simulink model "mcp4562"  (R2023b)
settings: Solver=VariableStepAuto  StartTime=0.0  StopTime=30  RelTol=1e-3
libraries: fl_lib x5, nesl_utility x3, ee_lib x1
settings Model: Creator=samuels  LastModifiedBy=samuels

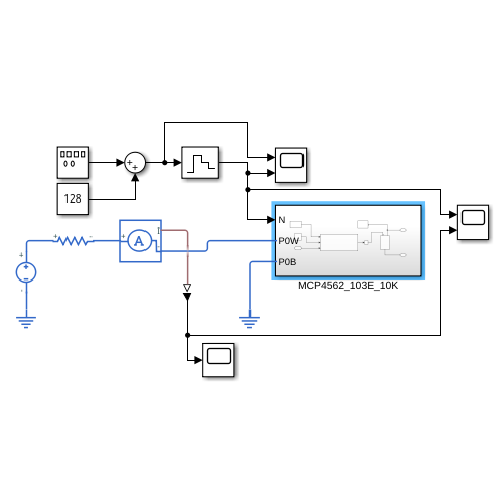
[thumbnail: Simulink's stored preview of the top-level diagram]
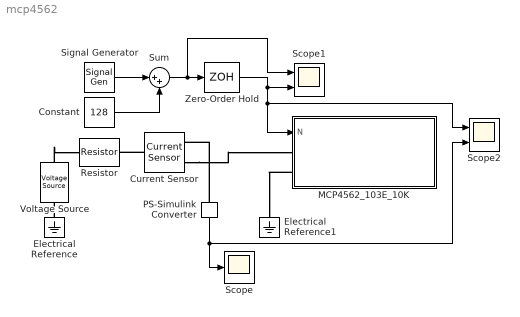
== system mcp4562 ==
  Constant : Constant  Value=128
  Current Sensor : fl_lib/Electrical/Electrical Sensors/Current Sensor
  Electrical Reference : fl_lib/Electrical/Electrical Elements/Electrical Reference
  Electrical Reference1 : fl_lib/Electrical/Electrical Elements/Electrical Reference
  MCP4562_103E_10K : Subsystem
  PS-Simulink Converter : nesl_utility/PS-Simulink Converter  PhysicalDomain=network_engine_domain  SubClassName=ps_output  LeftPortType=input  RightPortType=output  PseudoPeriodic=off  Frequencies=[]  VectorFormat=inherit  Unit=inherit  AffineConversion=off
  Resistor : fl_lib/Electrical/Electrical Elements/Resistor  R=100 Ohm  i_specify=off  i_priority=None  i=0 A  i_nominal_specify=off  i_nominal_unit=A  i_nominal_value=1  v_specify=off  v_priority=None  v=0 V  v_nominal_specify=off  v_nominal_unit=V  v_nominal_value=1
  Scope : Scope
  Scope1 : Scope  NumInputPorts=2
  Scope2 : Scope  NumInputPorts=2
  Signal Generator : SignalGenerator  WaveForm=sawtooth  Amplitude=128  Frequency=0.1
  Sum : Sum  Inputs=|++
  Voltage Source : ee_lib/Sources/Voltage Source  dc_voltage=1000 V  ac_voltage=0 V  ac_shift=0 rad  ac_frequency=60 Hz  noise_mode=ee.enum.sources.noise.Disabled  PSD=0 V^2/Hz  sample_time=1e-3 s  repeatability=ee.enum.sources.repeatability.NotRepeatable  user_seed=0  auto_seed=3499211588  i_specify=off  i_priority=None  i=0 A  i_nominal_specify=off  i_nominal_unit=A  i_nominal_value=1  v_specify=off  v_priority=None  v=0 V  v_nominal_specify=off  v_nominal_unit=V  v_nominal_value=1
  Zero-Order Hold : ZeroOrderHold  SampleTime=0.1
  wires:
  PS-Simulink Converter/1 -> Scope2/2, Scope/1
  Zero-Order Hold/1 -> Scope1/2, Scope2/1, MCP4562_103E_10K/1(N)
  Signal Generator/1 -> Sum/1
  Sum/1 -> Scope1/1, Zero-Order Hold/1
  Constant/1 -> Sum/2
  connections:
  Voltage Source/LConn1 -- Resistor/LConn1
  Electrical Reference/LConn1 -- Voltage Source/RConn1
  MCP4562_103E_10K/LConn2 -- Electrical Reference1/LConn1
  Current Sensor/LConn1 -- Resistor/RConn1
  Current Sensor/RConn2 -- MCP4562_103E_10K/LConn1
  PS-Simulink Converter/LConn1 -- Current Sensor/RConn1

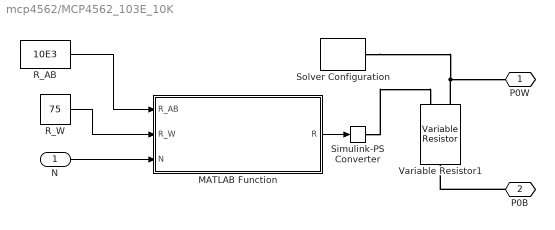
== system mcp4562/MCP4562_103E_10K ==
  N : Inport
  MATLAB Function : MATLAB Function  TreatAsAtomicUnit=on
  R_AB : Constant  Value=10E3
  R_W : Constant  Value=75
  Simulink-PS Converter : nesl_utility/Simulink-PS Converter  PhysicalDomain=network_engine_domain  SubClassName=ps_input  LeftPortType=input  RightPortType=output  PseudoPeriodic=off  Frequencies=[]  NoiseDistribution=none  NoiseParameters=[]  Unit=1  AffineConversion=off  FilteringAndDerivatives=provide  SimscapeFilterOrder=1  InputFilterTimeConstant=0.001  UdotUserProvided=0
  Solver Configuration : nesl_utility/Solver Configuration  PhysicalDomain=network_engine_domain  SubClassName=solver  LeftPortType=input  RightPortType=generic  Tones=[]  Harmonics=[]  SimulateNoise=off  Profile=off  UseLocalSampling=off  EnableSwitchedLinearOptims=on  FrequencyDomain=off  UseCCode=off  RelTol=0.001  AbsTol=0.001  MinStep=1e-09  ToWorkspace=off  RevertToSquareIcSolve=off  NumHomotopyIterations=100  PhasorMode=off  PhasorModeNumHarmonics=1  ConsistencySolver=NEWTON_XTOL_AFTER_FTOL  IndexReductionMethod=DerivativeReplacement  DoDC=off  ResidualTolerance=1e-09  ConsistencyTolSource=GLOBAL  ConsistencyAbsTol=0.001  ConsistencyRelTol=0.001  ConsistencyTolFactor=0.001  UseLocalSolver=off  LocalSolverChoice=NE_BACKWARD_EULER_ADVANCER  ResolveIndetEquations=on  FunctionEvalNumThread=1  LocalSolverSampleTime=0.001  DoFixedCost=off  MaxNonlinIter=3  MaxModeIter=2  ComputeImpulses=off  ImpulseIterations=2  LinearAlgebra=auto  LinearAlgebraNumThread=0  EquationFormulation=NE_TIME_EF  DelaysMemoryBudget=1024  AutomaticFiltering=on  FilteringTimeConstant=0.001  PartitionStorageMethod=AS_NEEDED  PartitionMemoryBudget=1024  PartitionMethod=ROBUST  MultibodyUseLocalSolver=off  MultibodyLocalSolverChoice=ODE1  MultibodyLocalSolverSampleTime=0.001
  Variable Resistor1 : fl_lib/Electrical/Electrical Elements/Variable Resistor  Rmin=0 Ohm  thermalEnable=false  thermal_mass=1 J/K  i_specify=off  i_priority=None  i=0 A  i_nominal_specify=off  i_nominal_unit=A  i_nominal_value=1  v_specify=off  v_priority=None  v=0 V  v_nominal_specify=off  v_nominal_unit=V  v_nominal_value=1  T_specify=off  T_priority=None  T=300 K  T_nominal_specify=off  T_nominal_unit=K  T_nominal_value=1
  P0W : PMIOPort  Side=Left
  P0B : PMIOPort  Port=2  Side=Left
  wires:
  R_AB/1 -> MATLAB Function/1(R_AB)
  R_W/1 -> MATLAB Function/2(R_W)
  N/1 -> MATLAB Function/3(N)
  MATLAB Function/1(R) -> Simulink-PS Converter/1
  connections:
  Variable Resistor1/LConn2 -- Solver Configuration/RConn1 -- P0W/RConn1
  P0B/RConn1 -- Variable Resistor1/RConn1
  Simulink-PS Converter/RConn1 -- Variable Resistor1/LConn1

== matlab function mcp4562/MCP4562_103E_10K/MATLAB Function ==
  data: R_AB input; R output; R_W input; N input
function R = MCP4562_103E_10K(R_AB, R_W, N)

% Based on register structure in device, N is allowed to be varied between
% 0 to 256. Setting N to 0 directly connects the wiper (W) to terminal B
% (no configurable resistance, only R_W). Increasing N increases the number
% of series resistors between the wiper and R_W.

R_S = R_AB/256; % Invidual series resistor is fraction of overall R_AB
R = R_S*N + R_W;
